simulink model "TORA_Linear"  (R2019b)
settings: Solver=VariableStepAuto  StartTime=0.0  StopTime=10.0  RelTol=1e-3
values from neighbouring files (symbols this model uses):
  Aa = [0 , 1 , 0 ,0 ... (first row only)    [main.m]
  Ba = [0 ... (first row only)    [main.m]
  Boolean_Flag_for_Controller = 1    [main.m]
  C = [1 0 0 0 ... (first row only)    [TORA_math2.m]    (also in main.m = [1 , 0 , 0 , 0)
  K = place(Aa , Ba , Pole_P)    [main.m]
  L_Value = place(Aa', C', desiredPoles)'    [main.m]
  stateEstimates = 1    [main.m]
  x0 = [0 0 0.01 0.01]'    [TORA_math2.m]    (also in main.m = [20*(ctoRadians) , 0 , 0.1, 0]')
  x_bar = [0 0 0 0]    [TORA_math2.m]    (also in main.m = [0 , 0 , 0 , 0]')
settings Model: Creator=don  LastModifiedBy=don

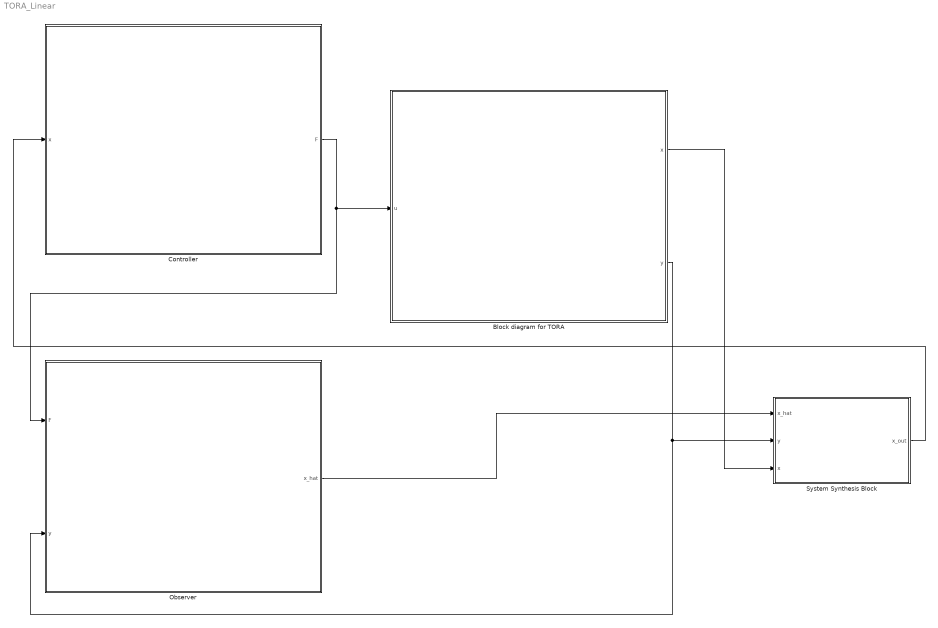
== system TORA_Linear ==
  Block diagram for TORA : Subsystem
  Controller : Subsystem
  Observer : Subsystem
  System Synthesis Block : Subsystem
  wires:
  Block diagram for TORA/2(y) -> Observer/2(y), System Synthesis Block/2(y)
  Controller/1(F) -> Block diagram for TORA/1(u), Observer/1(F)
  Observer/1(x_hat) -> System Synthesis Block/1(x_hat)
  Block diagram for TORA/1("x ") -> System Synthesis Block/3(x)
  System Synthesis Block/1(x_out) -> Controller/1(x)

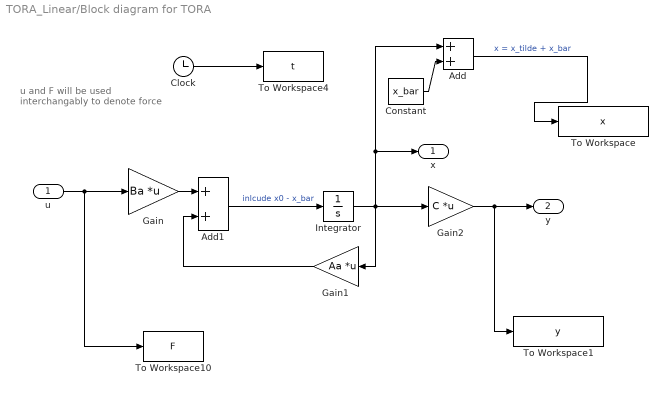
== system TORA_Linear/Block diagram for TORA ==
  note: u and F will be used
      | interchangably to denote force
  u : Inport
  Add : Sum
  Add1 : Sum
  Clock : Clock
  Constant : Constant  Value=x_bar
  Gain : Gain  Gain=Ba  Multiplication=Matrix(K*u)
  Gain1 : Gain  Gain=Aa  Multiplication=Matrix(K*u)
  Gain2 : Gain  Gain=C  Multiplication=Matrix(K*u)
  Integrator : Integrator  InitialCondition=x0-x_bar
  To Workspace : ToWorkspace  VariableName=x  SampleTime=-1
  To Workspace1 : ToWorkspace  VariableName=y  SampleTime=-1
  To Workspace10 : ToWorkspace  VariableName=F  SampleTime=-1
  To Workspace4 : ToWorkspace  VariableName=t  SampleTime=-1
  "x " : Outport  VectorParamsAs1DForOutWhenUnconnected=off
  y : Outport  Port=2  VectorParamsAs1DForOutWhenUnconnected=off
  wires:
  Integrator/1 -> Gain1/1, Add/1, "x "/1, Gain2/1
  Gain/1 -> Add1/1
  Add/1 -> To Workspace/1  "x = x_tilde + x_bar"
  u/1 -> Gain/1, To Workspace10/1
  Clock/1 -> To Workspace4/1
  Add1/1 -> Integrator/1  "inlcude x0 - x_bar"
  Gain2/1 -> To Workspace1/1, y/1
  Gain1/1 -> Add1/2
  Constant/1 -> Add/2

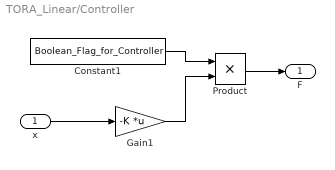
== system TORA_Linear/Controller ==
  x : Inport
  Constant1 : Constant  Value=Boolean_Flag_for_Controller
  Gain1 : Gain  Gain=-K  Multiplication=Matrix(K*u)
  Product : Product
  F : Outport
  wires:
  Product/1 -> F/1
  x/1 -> Gain1/1
  Gain1/1 -> Product/2
  Constant1/1 -> Product/1

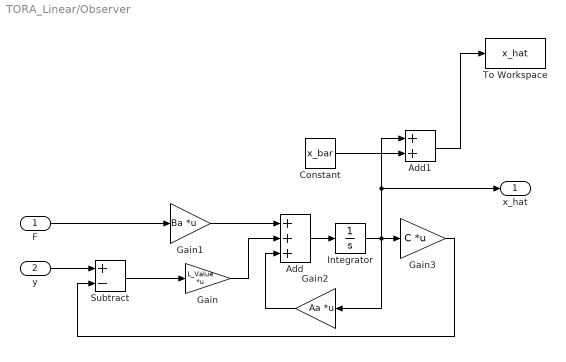
== system TORA_Linear/Observer ==
  F : Inport
  y : Inport  Port=2
  Add : Sum  Inputs=+++
  Add1 : Sum
  Constant : Constant  Value=x_bar
  Gain : Gain  Gain=L_Value  Multiplication=Matrix(K*u)
  Gain1 : Gain  Gain=Ba  Multiplication=Matrix(K*u)
  Gain2 : Gain  Gain=Aa  Multiplication=Matrix(K*u)
  Gain3 : Gain  Gain=C  Multiplication=Matrix(K*u)
  Integrator : Integrator
  Subtract : Sum  Inputs=+-
  To Workspace : ToWorkspace  VariableName=x_hat  SampleTime=-1
  x_hat : Outport  VectorParamsAs1DForOutWhenUnconnected=off
  wires:
  Add1/1 -> To Workspace/1
  Gain1/1 -> Add/1
  Integrator/1 -> Add1/1, x_hat/1, Gain2/1, Gain3/1
  y/1 -> Subtract/1
  F/1 -> Gain1/1
  Subtract/1 -> Gain/1
  Gain3/1 -> Subtract/2
  Gain2/1 -> Add/3
  Add/1 -> Integrator/1
  Constant/1 -> Add1/2
  Gain/1 -> Add/2

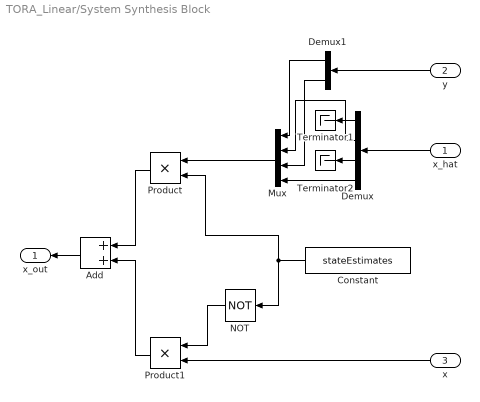
== system TORA_Linear/System Synthesis Block ==
  x_hat : Inport
  y : Inport  Port=2
  x : Inport  Port=3
  Add : Sum
  Constant : Constant  Value=stateEstimates
  Demux : Demux
  Demux1 : Demux  Outputs=2
  Mux : Mux
  NOT : Logic  Operator=NOT  IconShape=distinctive  AllPortsSameDT=off  OutDataTypeStr=boolean
  Product : Product
  Product1 : Product
  Terminator1 : Terminator
  Terminator2 : Terminator
  x_out : Outport
  wires:
  y/1 -> Demux1/1
  Demux/2 -> Mux/2
  Constant/1 -> NOT/1, Product/2
  NOT/1 -> Product1/1
  Demux/3 -> Terminator2/1
  Product1/1 -> Add/2
  x_hat/1 -> Demux/1
  Demux1/1 -> Mux/1
  x/1 -> Product1/2
  Demux/1 -> Terminator1/1
  Product/1 -> Add/1
  Add/1 -> x_out/1
  Demux1/2 -> Mux/3
  Mux/1 -> Product/1
  Demux/4 -> Mux/4
